simulink model "Raw_read_SerialFrame"  (R2025b)
settings: Solver=FixedStepAuto  StartTime=0.0  StopTime=inf  FixedStep=0.0002  RelTol=1e-3
undefined symbols (not defined in the file or in its folder): CR, LF
libraries: instrumentseriallib x2, svdutilitieslib x2
settings Model: VariantFading=off  Creator=Akkarasaknarong  LastModifiedBy=Akkarasaknarong

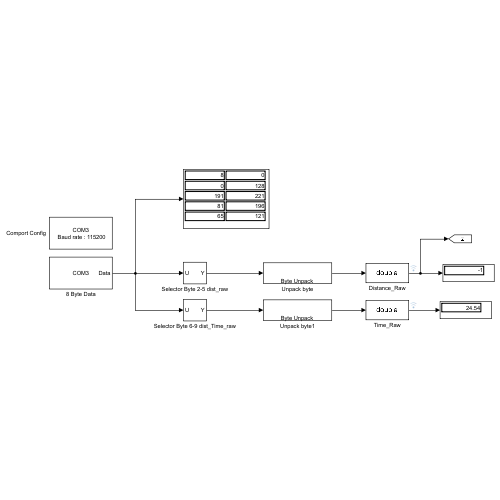
[thumbnail: Simulink's stored preview of the top-level diagram]
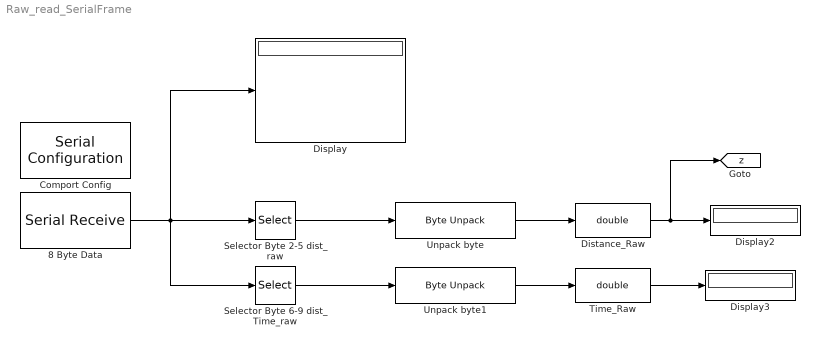
== system Raw_read_SerialFrame ==
  8 Byte Data : instrumentseriallib/Serial Receive  Priority=1  PortSel=COM3  Port=COM3  ComPort=COM3  DataType=uint8  SaveDataType=uint8  ToggleHeader=on  Header=[170 85]  ToggleDataSize=on  DataSize=[10 1]  ToggleTerminator=off  Terminator=CR/LF ('\r\n')  CustomTerminator=[]  InputFormat=Column major  EnableBlockingMode=on  ActionDataUnavailable=Output last received value  ActionWhenDataUnavailable=Output last received value  CustomValue=-50  SampleTime=0.0002  SimulateUsing=Interpreted execution  BlockInModel=on  aMode=1  LibraryInUse=instrumentlib
      settings: LibrarySourceBlock=embeddedtargetslib/Host Communication/Serial Receive
  Comport Config : instrumentseriallib/Serial Configuration  Priority=-200000  PortSel=COM3  Port=COM3  ComPort=COM3  BaudRate=115200  DataBits=8  Parity=none  StopBits=1  ByteOrder=little-endian  FlowControl=none  Timeout=10  SimulateUsing=Interpreted execution  BlockInModel=on  aMode=1
      settings: LibrarySourceBlock=embeddedtargetslib/Host Communication/Serial Configuration
  Display : Display
  Display2 : Display
  Display3 : Display
  Distance_Raw : DataTypeConversion  OutDataTypeStr=double  SaturateOnIntegerOverflow=off  RndMeth=Floor
  Selector Byte 2-5 dist_raw : Selector  InputPortWidth=10  IndexOptions=Index vector (dialog)  Indices=[2 3 4 5]  OutputSizes=1
  Selector Byte 6-9 dist_Time_raw : Selector  InputPortWidth=10  IndexOptions=Index vector (dialog)  Indices=[6 7 8 9]  OutputSizes=1
  Time_Raw : DataTypeConversion  OutDataTypeStr=double  SaturateOnIntegerOverflow=off  RndMeth=Floor
  Unpack byte : svdutilitieslib/Byte Unpack  dimensions={[1]}  datatypes={'single'}  byteAlign=1  blockPlatform=arduinoert
      settings: LibrarySourceBlock=mcblib/Signal Management/Byte Unpack
  Unpack byte1 : svdutilitieslib/Byte Unpack  dimensions={[1]}  datatypes={'single'}  byteAlign=1  blockPlatform=arduinoert
      settings: LibrarySourceBlock=mcblib/Signal Management/Byte Unpack
  tag scope: z=global
  wires:
  Selector Byte 6-9 dist_Time_raw/1 -> Unpack byte1/1
  8 Byte Data/1 -> Display/1, Selector Byte 2-5 dist_raw/1, Selector Byte 6-9 dist_Time_raw/1
  Unpack byte1/1 -> Time_Raw/1
  Unpack byte/1 -> Distance_Raw/1
  Selector Byte 2-5 dist_raw/1 -> Unpack byte/1
  Distance_Raw/1 -> [z], Display2/1
  Time_Raw/1 -> Display3/1
